simulink model "Project_microgrid"  (R2019b)
settings: Solver=FixedStepAuto  StartTime=0.0  StopTime=0.3  RelTol=1e-3
undefined symbols (not defined in the file): D1, D11, Delta, DiscIntNeverNeededParam, find_system, Hydride, Metal, Nickel
libraries: powerlib x108, powerlib_meascontrol x31, sps_avr x14, simulink_extras x4, simulink x3, spsDieselMotorModel x2, electricdrivelib x1, re_lib x1
(part 1 of 5)
settings Model: Creator=mdeat  LastModifiedBy=md ether
settings OptimizationCC: DefaultParameterBehavior=Inlined  EnhancedBackFolding=on  PassReuseOutputArgsAs=Individual arguments  ZeroExternalMemoryAtStartup=off  ZeroInternalMemoryAtStartup=off  MaxStackSize=64  OptimizeBlockOrder=speed  DifferentSizesBufferReuse=on  OptimizationCustomize=off  EfficientTunableParamExpr=on
settings DebuggingCC: ParameterTunabilityLossMsg=error
settings HardwareCC: ProdBitPerPointer=32  ProdBitPerSizeT=32  ProdBitPerPtrDiffT=32  ProdLargestAtomicInteger=Long  ProdLargestAtomicFloat=Double  ProdWordSize=32  ProdHWDeviceType=ARM Compatible->ARM Cortex
settings SFSimCC: MATLABDynamicMemAlloc=off  CustomCodeUndefinedFunction=UseInterfaceOnly
settings RTWCC: SystemTargetFile=ert.tlc  TemplateMakefile=ert_default_tmf  GenerateReport=on  Toolchain=Android SDK/NDK Tools  IncludeHyperlinkInReport=on  LaunchReport=on  GenerateTraceInfo=on  GenerateTraceReport=on  GenerateTraceReportSl=on  GenerateTraceReportSf=on  GenerateTraceReportEml=on
settings CodeAppCC: ForceParamTrailComments=on  IgnoreCustomStorageClasses=off  OperatorAnnotations=on  SimulinkDataObjDesc=on  SFDataObjDesc=on  InsertBlockDesc=on
settings ERTTargetCC: SupportContinuousTime=on  InlinedParameterPlacement=NonHierarchical  ERTCustomFileTemplate=example_file_process.tlc

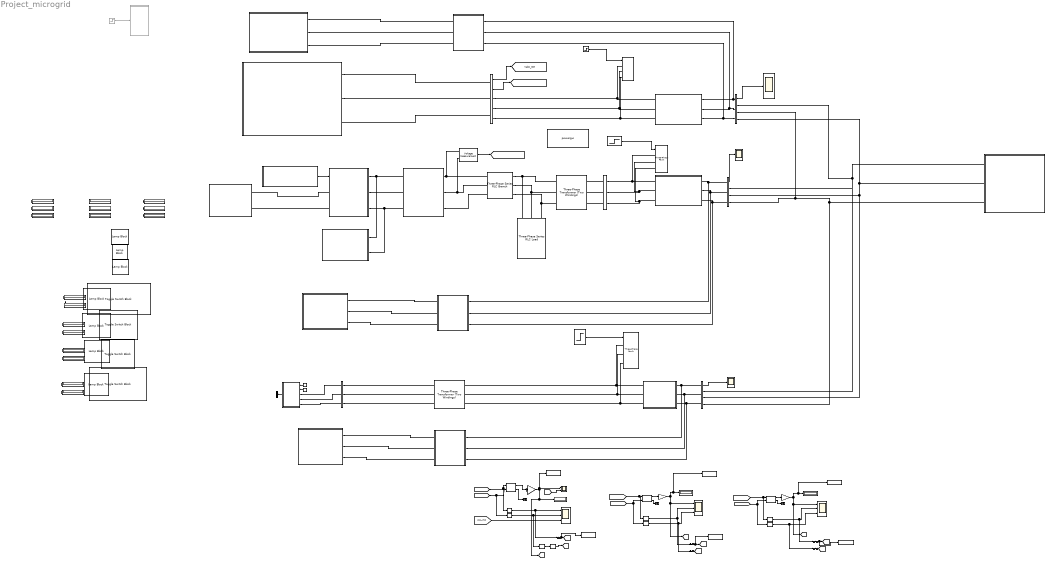
== system Project_microgrid ==
  note: Diesle Generator Output
  note: Wind Plant Output
  note: PV Output
  note: Fault Status
  note: Solar Power
  note: Solar Voltage
  note: Gen. Voltage
  note: Wind Power
  note: Gen. Current
  note: Current Power Status
  note: Gen. Power
  note: Solar Current
  note: Wind Current
  note: Wind Voltage
  note: PV Bus Fault
  note: Wind Bus Fault
  note: Generator Bus Fault
  note: Branch Status in Grid System
  note: Bus 1 Current
  note: Bus 1 Voltage
  note: Bus 2 Current
  note: Bus 2 Voltage
  note: Bus 3 Current
  note: Bus 3 Voltage
  note: Bus 4 Current
  note: Bus 4 Voltage
  " 2.2MWGenerator Backup" : Subsystem
  10 kvar Filter : powerlib/Elements/Three-Phase Series RLC Load  LConnTagsString=A|B|C  Configuration=Y (grounded)  NominalVoltage=240  Vabc=[1e3 1e3 1e3]  Vabcp=[1e3 1e3 1e3]  NominalFrequency=50  UnbalancedPower=off  ActivePower=10e3/100  InductivePower=0  CapacitivePower=10e3  Pabc=[10e3 9e3 11e3]  QLabc=[100 90 110]  QCabc=[100 90 110]  Pabcp=[10e3 9e3 11e3]  QLabcp=[100 90 110]  QCabcp=[100 90 110]  Measurements=None  LoadType=constant Z  mask(Three-Phase Series RLC Load){}
      settings: SourceProductName=Simscape Electrical
  100KW PV Backup : Subsystem
  260V / 25 kV : powerlib/Elements/Three-Phase Transformer (Two Windings)  Winding1Connection=Yg  Winding2Connection=Delta (D1)  CoreType=Three single-phase transformers  SetSaturation=off  Hysteresis=off  DataFile='hysteresis'  SetInitialFlux=off  Measurements=None  UNITS=pu  NominalPower=[7500 , 50 ]  Winding1=[ 25e3 , 0.001 , 0.03 ]  Winding2=[ 260 , 0.001 , 0.03 ]  Rm=500  Lm=500  L0=0.5  Saturation=[ 0,0 ; 0.0024,1.2 ; 1.0,1.52 ]  InitialFluxes=[ 0.8 , -0.8 , 0.7 ]  BreakLoop=off  DiscreteSolver=Trapezoidal iterative  DataType=off  TransfoNumber=0  mask(Three-Phase Transformer (Two Windings)){}
      settings: SourceProductName=Simscape Electrical
  "575 V/ 25 kV " : powerlib/Elements/Three-Phase Transformer (Two Windings)  Winding1Connection=Delta (D11)  Winding2Connection=Yg  CoreType=Three single-phase transformers  SetSaturation=off  Hysteresis=off  DataFile='hysteresis'  SetInitialFlux=off  Measurements=None  UNITS=pu  NominalPower="[2.5e6*5  60]"  Winding1=[25e3 , 0.025/30 , 0.025]  Winding2=[ 575, 0.025/30 , 0.025]  Rm=500  Lm=inf  L0=0.5  Saturation=[ 0,0 ; 0.0024,1.2 ; 1.0,1.52 ]  InitialFluxes=[ 0.8 , -0.8 , 0.7 ]  BreakLoop=off  DiscreteSolver=Trapezoidal iterative  DataType=off  TransfoNumber=0  mask(Three-Phase Transformer (Two Windings)){}
      settings: SourceProductName=Simscape Electrical
  600 KW Wind Backup2 : Subsystem
  Battery : Subsystem
  "Boost Conveter " : Subsystem
  Bus Selector : BusSelector  OutputSignals=Vdc_V,wr_pu,PQ_pu.P_pu,PQ_pu.Q_pu
  Constant : Constant  Value=15
  Constant1 : Constant  Value=0
  "Diesel Generator Bus " : powerlib/Measurements/Three-Phase V-I Measurement  VoltageMeasurement=phase-to-ground  SetLabelV=off  LabelV=Vabc  Vpu=off  VpuLL=off  CurrentMeasurement=yes  SetLabelI=off  LabelI=Iabc  Ipu=off  Pbase=100e6  Vbase=500e3  OutputType=Complex  PhasorSimulation=off  PSBequivalent=0
      settings: SourceProductName=Simscape Electrical
  Diesel Generator Bus 1 : powerlib/Measurements/Three-Phase V-I Measurement  VoltageMeasurement=no  SetLabelV=off  LabelV=Vabc  Vpu=off  VpuLL=off  CurrentMeasurement=yes  SetLabelI=off  LabelI=Iabc  Ipu=off  Pbase=100e6  Vbase=500e3  OutputType=Complex  PhasorSimulation=off  PSBequivalent=0
      settings: SourceProductName=Simscape Electrical
  Diesle Generator : Subsystem
  Grid : Scope  NumInputPorts=3
  Grid System : Subsystem
  Grid1 : Scope  NumInputPorts=3
  Grid2 : Scope  NumInputPorts=3
  Inveter : Subsystem
  Lamp{,1..6} (7 alike) : LampBlock
  MATLAB Function : MATLAB Function  Commented=on  TreatAsAtomicUnit=on
  "MPPT Controler " : Subsystem
  P (kW){,1..19} (20 alike) : Display
      settings: Format=bank  Decimation=2000
  PV Bus : powerlib/Measurements/Three-Phase V-I Measurement  VoltageMeasurement=phase-to-ground  SetLabelV=on  LabelV=Vabc_PV  Vpu=off  VpuLL=off  CurrentMeasurement=yes  SetLabelI=on  LabelI=Iabc_PV  Ipu=off  Pbase=100e6  Vbase=500e3  OutputType=Magnitude  PhasorSimulation=off  PSBequivalent=0
      settings: SourceProductName=Simscape Electrical
  PV Bus 1 : powerlib/Measurements/Three-Phase V-I Measurement  VoltageMeasurement=phase-to-ground  SetLabelV=off  LabelV=Vabc  Vpu=off  VpuLL=off  CurrentMeasurement=no  SetLabelI=off  LabelI=Iabc  Ipu=off  Pbase=100e6  Vbase=500e3  OutputType=Complex  PhasorSimulation=off  PSBequivalent=0
      settings: SourceProductName=Simscape Electrical
  "PV System " : Subsystem
  P_B1 : Scope  NumInputPorts=2
  Power (Positive-Sequence) : powerlib_meascontrol/Measurements/Power (Positive-Sequence)  Freq=60  Vinit=[0, 0]  Iinit=[0, 0]  Ts=0.0001
      settings: SourceProductName=Simscape Electrical  SourceProductBaseCode=PS
  Power (Positive-Sequence)1 : powerlib_meascontrol/Measurements/Power (Positive-Sequence)  Freq=60  Vinit=[0, 0]  Iinit=[0, 0]  Ts=0.0001
      settings: SourceProductName=Simscape Electrical  SourceProductBaseCode=PS
  Power (Positive-Sequence)2 : powerlib_meascontrol/Measurements/Power (Positive-Sequence)  Freq=60  Vinit=[0, 0]  Iinit=[0, 0]  Ts=0.0001
      settings: SourceProductName=Simscape Electrical  SourceProductBaseCode=PS
  Relay G : Subsystem
  Relay PV : Subsystem
  Relay W : Subsystem
  Scope2 : Scope
  Scope3 : Scope
  Scope4 : Scope
  Selector{,1..5} (6 alike) : Selector  InputPortWidth=3  IndexOptions=Index vector (dialog)  Indices=[1]  OutputSizes=1
  Sqrt{,1..5} (6 alike) : Sqrt  SaturateOnIntegerOverflow=on
  Square{,1..5} (6 alike) : Math  Operator=square  SignedPower=off  SaturateOnIntegerOverflow=on
  Step : Step  Commented=on  Time=0.5  After=5  SampleTime=0
  Step1 : Step  Time=0.25  SampleTime=0
  Step2 : Step  Time=0.05  SampleTime=0
  Step3 : Step  Time=0.2  SampleTime=0
  Switching Sustem : Subsystem
  Switching Sustem1 : Subsystem
  Switching Sustem3 : Subsystem
  TX Line Parameter : powerlib/Elements/Three-Phase Series RLC Branch  LConnTagsString=A|B|C  RConnTagsString=A|B|C  BranchType=RL  Resistance=500e-6*377/50/2  Inductance=500e-6/2  Capacitance=inf  Measurements=None
      settings: SourceProductName=Simscape Electrical
  Terminator1 : Terminator
  Terminator2 : Terminator
  Terminator3 : Terminator
  Three-Phase Fault1 : powerlib/Elements/Three-Phase Fault  InitialStates=[0 0 0]  FaultA=on  FaultB=on  FaultC=on  GroundFault=on  SwitchTimes="[1/60  5/60]"  External=on  SwitchStatus=NaN  FaultResistance=0.1  GroundResistance=0.01  SnubberResistance=1e6  SnubberCapacitance=inf  Measurements=None
      settings: SourceProductName=Simscape Electrical
  Three-Phase Fault2 : powerlib/Elements/Three-Phase Fault  InitialStates=[0 0 0]  FaultA=on  FaultB=on  FaultC=on  GroundFault=on  SwitchTimes="[1/60  5/60]"  External=on  SwitchStatus=NaN  FaultResistance=0.1  GroundResistance=0.01  SnubberResistance=1e6  SnubberCapacitance=inf  Measurements=None
      settings: SourceProductName=Simscape Electrical
  Three-Phase Fault3 : powerlib/Elements/Three-Phase Fault  InitialStates=[0 0 0]  FaultA=on  FaultB=on  FaultC=on  GroundFault=on  SwitchTimes="[1/60  5/60]"  External=on  SwitchStatus=NaN  FaultResistance=0.1  GroundResistance=0.01  SnubberResistance=1e6  SnubberCapacitance=inf  Measurements=None
      settings: SourceProductName=Simscape Electrical
  To Workspace : ToWorkspace  VariableName=PV_P  SaveFormat=Timeseries  SampleTime=-1
  To Workspace1 : ToWorkspace  VariableName=PV_V  SaveFormat=Timeseries  SampleTime=-1
  To Workspace2 : ToWorkspace  VariableName=W_P  SaveFormat=Timeseries  SampleTime=-1
  To Workspace3 : ToWorkspace  VariableName=W_V  SaveFormat=Timeseries  SampleTime=-1
  To Workspace4 : ToWorkspace  VariableName=G_P  SaveFormat=Timeseries  SampleTime=-1
  To Workspace5 : ToWorkspace  VariableName=G_V  SaveFormat=Timeseries  SampleTime=-1
  Toggle Switch{,1..3} (4 alike) : ToggleSwitchBlock
      settings: Values={{'Off', 'On'}, [0 1]}
  Vdc 1 : powerlib/Measurements/Voltage Measurement  Tag=PoWeRsYsTeMmEaSuReMeNt  PhasorSimulation=off  OutputType=Magnitude  PSBequivalent=0
      settings: SourceProductName=Simscape Electrical
  W : Gain  Gain=1/1000
  W1 : Gain  Gain=33.44
  W2kW : Gain  Gain=1/1000
  W2kW1 : Gain  Gain=1/1000
  Wind Bus : powerlib/Measurements/Three-Phase V-I Measurement  VoltageMeasurement=phase-to-ground  SetLabelV=on  LabelV=Vabc_Wind  Vpu=off  VpuLL=off  CurrentMeasurement=yes  SetLabelI=on  LabelI=Iabc_Wind  Ipu=off  Pbase=5*2e6/0.9  Vbase=575  OutputType=Complex  PhasorSimulation=off  PSBequivalent=0
      settings: SourceProductName=Simscape Electrical
  Wind Bus 1 : powerlib/Measurements/Three-Phase V-I Measurement  VoltageMeasurement=phase-to-ground  SetLabelV=off  LabelV=Vabc  Vpu=off  VpuLL=off  CurrentMeasurement=no  SetLabelI=off  LabelI=Iabc  Ipu=off  Pbase=100e6  Vbase=500e3  OutputType=Complex  PhasorSimulation=off  PSBequivalent=0
      settings: SourceProductName=Simscape Electrical
  Wind Turbine Type 4 : Subsystem  LoadFcn=%find_system(gcs,'FollowLinks', 'on', 'LookUnderMasks', 'all');  mask(Wind Turbine: Model 7){Nb_wt=5, ShowParameters=Generator data for 1 wind turbine, nom=[2e6/0.9 730 60], Reactances=[ 1.305, 0.296, 0.252, 0.474,  0.243,  0.18 ], Time_constants=[  4.49  0.0681  0.0513  ], Resistance=0.006, mec=[0.62 0.01 1], init=[ 0  0  0  0  0  0  0  0  1 ], Vnom=575, Imax_grid_conv=1.1, RL_grid=[ 0.15 0.15/50], C_var_filter1=150e3, Vdc_nom=1100, C_DClink1=90000e-6, L_R_Boost=[0.0012     5e-3], Pmec1=2e6, wind_speed_CpMax=11, wind0=11, DisplayTurbChar=off, H_WT=4.32, Ksh=0.3, D_mutual=1.5, w_wt0=1, torque0=1, Kdc=[1.1   27.5], Ki_var_reg=0.05, Ki_volt_reg=2, Kgrid_side_cur_reg=[1  50], Kspeed=[5 1], Kboost_cur_reg=[0.025 100], Kp_pitch=15, Kcompensation=[1.5  6], Kfield=[10  20], pitch_max=27, pitch_rate=10, Ts=2e-6}
      mask prompts: Nb_wt "Number of wind turbines:"; ShowParameters "Display:"; nom "Nom. power, L-L volt. and freq.: [Pn (VA), Vn (Vrms), fn (Hz)]"; Reactances "Reactances [Xd Xd' Xd'' Xq Xq'' Xl] (p.u.):"; Time_constants "Time constants [Tdo' Tdo'' Tq''] (s):"; Resistance "Resistance Rs (p.u.):"; mec "Inertia constant, friction factor, and pairs of poles: [ H(s)  F(p.u.)  p ]"; init "Initial conditions: [dw(%) th(deg) ia,ib,ic(pu) pha,phb,phc(deg) Vf(pu)]:"; Vnom "Grid-side converter nominal AC voltage (V):"; Imax_grid_conv "Grid-side converter maximum AC current (pu based on generator power and converter nominal AC voltage):"; RL_grid "Grid-side coupling inductor [ L(pu) R(pu),pu based on generator power and converter nominal AC voltage] :"; C_var_filter1 "Line filter capacitor (Q=50) (var):"; Vdc_nom "Nominal DC bus voltage (V)"; C_DClink1 "DC bus capacitor (F):"; L_R_Boost "Boost converter inductance [L(H) R(ohm)]:"; Pmec1 "Nominal mechanical output power (W):"; wind_speed_CpMax "Wind speed at nominal speed and at Cp max (must be between 6 m/s and 30 m/s) (m/s):"; wind0 "Initial wind speed (m/s):"; DisplayTurbChar "Display wind turbine power characteristics:"; H_WT "Wind turbine inertia constant H (s):"; Ksh "Shaft spring constant refer to high-speed shaft (pu of nominal mechanical torque/rad):"; D_mutual "Shaft mutual damping (pu of nominal mechanical torque/pu dw):"; w_wt0 "Turbine initial speed (pu of nominal speed):"; torque0 "Initial output torque (pu of nominal mechanical torque):"; Kdc "DC bus voltage regulator gains [Kp Ki]:"; Ki_var_reg "Grid-side converter var regulator gain [ Ki]:"; Ki_volt_reg "Grid-side converter voltage regulator gain [ Ki]:"; Kgrid_side_cur_reg "Grid-side converter current regulator gains [Kp Ki]:"; Kspeed "Speed regulator gains [Kp Ki]:"; Kboost_cur_reg "Boost inductor current regulator gains [Kp Ki]:"; Kp_pitch "Pitch controller gain [Kp]:"; Kcompensation "Pitch compensation gains [Kp Ki]:"; Kfield "Field excitation gains [Kp Ki]:"; pitch_max "Maximum pitch angle (deg):"; pitch_rate "Maximum rate of change of pitch angle (deg/s)"; Ts "Sample time (s):"
      mask help: This block implements a model of a variable speed pitch controlled wind turbine using a synchronous generator.
      mask init:
      | %Generator data
      | Pnom=nom(1)*Nb_wt;
      | Vnom_gen=nom(2);
      | Fnom=nom(3);
      | Xd=Reactances(1);
      | Xd1=Reactances(2);
      | Xd2=Reactances(3);
      | Xq=Reactances(4);
      | Xq2=Reactances(5);
      | Xl=Reactances(6);
      | Tdo1=Time_constants(1);
      | Tdo2=Time_constants(2);
      | Tq2=Time_constants(3);
      | H=mec(1);
      | F=mec(2);
      | p=mec(3);
      | 
      | % Converters data
      | L_RL=RL_grid(1);
      | R_RL=RL_grid(2);
      | L_Boost=L_R_Boost(1)/Nb_wt;
      | R_Boost=L_R_Boost(2)/Nb_wt;
      | Q_filter=50;
      | C_DClink=C_DClink1*Nb_wt;
      | C_var_filter=C_var_filter1*Nb_wt;
      | 
      | % Controller data
      | Freq_filter=10000;   %Hz
      | Zeta_filter=0.707;
      | Kp_dc=Kdc(1);
      | Ki_dc=Kdc(2);
      | Kp_grid_side_cur_reg=Kgrid_side_cur_reg(1);
      | Ki_grid_side_cur_reg=Kgrid_side_cur_reg(2);
      | Kp_speed=Kspeed(1);
      | Ki_speed=Kspeed(2);
      | Kp_boost_cur_reg=Kboost_cur_reg(1);
      | Ki_boost_cur_reg=Kboost_cur_reg(2);
      | Kp_compensation=Kcompensation(1);
      | Ki_compensation=Kcompensation(2);
      | Kp_field=Kfield(1);
      | Ki_field=Kfield(2);
      | Mod_index_max=1.1;
      | T_speed=5;      %Speed reference time constant (s)
      | Iq_ref_limit_time_constant=0.3; %(s)
      | Current_reg_output_limit=1.1;   %(pu)
      | Var_reg_output_hi_limit=1.1;    %(pu)
      | Var_reg_output_low_limit=0.9;   %(pu)
      | Pitch_time_constant=0.01;       %(s)
      | Vf_limit=10;    %Field voltage limit (pu)
      | Flux_meas_time_constant=1*(1/Fnom); %(s)
      | Freq_sawtooth=2000; %Hz, Boost converter
      | Freq_PWM=3000; %Hz, Inverter
      | Ts_snub=50e-6;  %Sample time to compute snubber resistance
      | 
      | 
      | % Turbine data
      | Pmec=Pmec1*Nb_wt;
      | c1 = 0.6450;
      | c2 = 116;
      | c3 = .4;
      | c4 = 5;
      | c5 = 21;
      | c6 = .00912;  % Set Pmin in stall condition (does not vary with wind_speed_Pmax)
      | c7 = .08;
      | c8 = .035;
      | theta=0;
      | CpMax=.5;
      | lambda_CpMax=9.9495;
      | 
      | c1_c8=[c1 c2 c3 c4 c5 c6 c7 c8];
      |   
      | 
      | %   Cp = c1*(c6*lambda + (-c4 - c3*(2.5 + theta) + c2*(1/(lambda + ...
      | %   c7*(2.5 + theta)) - c8/(1 + (2.5 + theta)^3)))/exp(c5*(1/(lambda + ...
      | %   c7*(2.5 + theta)) - c8/(1 + (2.5 + theta)^3))))
      | 
      | 
      |         %%%%%%%%%%%%%%%%%%%%%%%%%%%%%%%%%%%%%%%%%%%%%%%%%%%%%%%%%%%%%%%%%%%%%%%%%%%
      |         % Operation at Cp max
      |         %%%%%%%%%%%%%%%%%%%%%%%%%%%%%%%%%%%%%%%%%%%%%%%%%%%%%%%%%%%%%%%%%%%%%%%%%%%
      |         
      |         rated_omegar=1;
      |         omegar = rated_omegar;
      |         
      |         % Enforce boundaries on wind speed
      |         % A warning could be displayed
      |         if wind_speed_CpMax < 6
      |             wind_speed_CpMax=6;
      |             disp('Warning: Wind speed at nominal speed and at Cp max has been set to 6 m/s')
      |         end
      |         if wind_speed_CpMax > 30
      |             wind_speed_CpMax=30;
      |             disp('Warning: Wind speed at nominal speed and at Cp max has been set to 30 m/s')
      |         end
      | 
      |         K1=lambda_CpMax/omegar*wind_speed_CpMax;
      |         
      |         % Calculation of K2 needed to get P equal to the requested value at
      |         % Cp max for the requested wind speed
      |         
      |         Prated=Pmec;
      |         P_rated_omegar_theta_zero=0.75;
      |         
      |         K2 = P_rated_omegar_theta_zero*Prated/(wind_speed_CpMax^3*CpMax);
      |         
      |         K1_K2=[K1 K2];
      |         
      |         %%%%%%%%%%%%%%%%%%%%%%%%%%%%%%%%%%%%%%%%%%%%%%%%%%%%%%%%%%%%%%%%%%%%%%%%%%%
      |         % End of calculation for operation at Cp max
      |         %%%%%%%%%%%%%%%%%%%%%%%%%%%%%%%%%%%%%%%%%%%%%%%%%%%%%%%%%%%%%%%%%%%%%%%%%%%
      |         
      | 
      | %%%%%%%%%%%%%%%%%%%%%%%%%%%%%%%%%%%%%%%%%%%%%%%%%%%%%%%%%%%%%%%%%%%%%%%%%%%
      | % Plot turbine characteristics
      | %%%%%%%%%%%%%%%%%%%%%%%%%%%%%%%%%%%%%%%%%%%%%%%%%%%%%%%%%%%%%%%%%%%%%%%%%%% 
      | 
      | DisplayTurbChar=get_param(gcb,'DisplayTurbChar');
      | if strcmp(DisplayTurbChar,'on')
      |     vect_theta = 0:2:30;
      |     
      |     vect_lambda = 1:0.2:30;
      |     
      |     clear Cp;
      |     
      |     for i=1:length(vect_theta)
      |      for j=1:length(vect_lambda)
      |                 Cp(i,j) = c1*(c6*vect_lambda(j) + (-c4 - c3*(2.5 + vect_theta(i)) + c2*(1/(vect_lambda(j) + ...
      |                 c7*(2.5 + vect_theta(i))) - c8/(1 + (2.5 + vect_theta(i))^3)))/exp(c5*(1/(vect_lambda(j) + ...
      |                 c7*(2.5 + vect_theta(i))) - c8/(1 + (2.5 + vect_theta(i))^3))));
      |      end
      |     end
      | 
      |     figure(1);
      |     clf;
      |     hold on;
      | 
      |     plot(vect_lambda, Cp);
      |     axis([0, 25, 0, .6]);
      |     title('Wind Turbine Cp Characteristic (pitch angle increases by step of 2 deg.)');
      |     ylabel('Cp');
      |     set(gca,'ytick',[0 .1 .2 .3 .4 .5 .6]);
      |     xlabel('Lambda');
      |     grid on;
      |     text(10.1,0.51,'Pitch angle 0 degree');
      | 
      |     hold off
      |     
      |     % Plot of the wind turbine mechanical power output (pu) lambda and Cp
      |     % characteristics against wind speed (m/s) for a range of theta.
      |     
      |     wind_speed_range = [1,.2,30];
      |     vect_wind_speed = 1:0.2:30;
      |     
      |     clear lambda;
      |     clear Cp;
      |     clear P;
      | 
      |     for i=1:length(vect_theta)
      |         for j=1:length(vect_wind_speed)
      |             lambda(i,j) = K1*omegar/vect_wind_speed(j);
      |             Cp(i,j) = c1*(c6*lambda(i,j) + (-c4 - c3*(2.5 + vect_theta(i)) + c2*(1/(lambda(i,j) + ...
      |             c7*(2.5 + vect_theta(i))) - c8/(1 + (2.5 + vect_theta(i))^3)))/exp(c5*(1/(lambda(i,j) + ...
      |             c7*(2.5 + vect_theta(i))) - c8/(1 + (2.5 + vect_theta(i))^3))));
      |             P(i,j) = K2/Prated*vect_wind_speed(j)^3*Cp(i,j);
      |         end
      |     end
      |     
      |     
      |     figure(2);
      |     clf;
      |     hold on
      |     
      |     subplot(3,1,1);
      |     plot(vect_wind_speed, P);
      |     axis([0, 35, 0, 1.5]);
      |     title('Wind Turbine Characteristics (w = 1 pu, pitch angle increases by step of 2 deg.)');
      |     ylabel('P (pu)');
      |     set(gca,'ytick',0:.5:4);
      |     grid on;
      |     
      |     subplot(3,1,2);
      |     plot(vect_wind_speed, lambda);
      |     axis([0, 35, 0, 20]);
      |     ylabel('Lambda');
      |     grid on;
      |     
      |     subplot(3,1,3)
      |     plot(vect_wind_speed, Cp);
      |     axis([0, 35, 0, .6]);
      |     xlabel('Wind Speed (m/s)');
      |     ylabel('Cp');
      |     set(gca,'ytick',[0 .1 .2 .3 .4 .5 .6]);
      |     grid on;
      | 
      |     hold off
      |     set_param(gcb,'DisplayTurbChar','off')
      |     
      | end
      mask TypeOptions ShowParameters: Generator data for 1 wind turbine | Converters data for 1 wind turbine | Turbine data for 1 wind turbine | Drive train data for 1 wind turbine | Control parameters for 1 wind turbine
      mask Callback ShowParameters:
      | BlockName=getfullname(gcb);
      | %
      | Param_Show=get_param(BlockName,'ShowParameters');
      | Param_DisplayTurbChar=get_param(BlockName,'DisplayTurbChar');
      | 
      | p_mask{3}='off';p_mask{4}='off';p_mask{5}='off';
      | p_mask{6}='off';p_mask{7}='off';p_mask{8}='off';p_mask{9}='off';
      | p_mask{10}='off';p_mask{11}='off';p_mask{12}='off';p_mask{13}='off';
      | p_mask{14}='off';p_mask{15}='off';p_mask{16}='off';p_mask{17}='off';
      | p_mask{18}='off';p_mask{19}='off';p_mask{20}='off';p_mask{21}='off';
      | p_mask{22}='off';p_mask{23}='off';p_mask{24}='off';p_mask{25}='off';
      | p_mask{26}='off';p_mask{27}='off';p_mask{28}='off';p_mask{29}='off';
      | p_mask{30}='off';p_mask{31}='off';p_mask{32}='off';p_mask{33}='off';
      | p_mask{34}='off';p_mask{35}='off';
      | 
      | switch Param_Show
      | 	case 'Generator data for 1 wind turbine'
      | 		p_mask{3}='on';p_mask{4}='on';p_mask{5}='on';
      |         p_mask{6}='on';p_mask{7}='on';p_mask{8}='on';
      |     case 'Converters data for 1 wind turbine'
      | 		p_mask{9}='on';p_mask{10}='on';p_mask{11}='on';
      |         p_mask{12}='on';p_mask{13}='on';p_mask{14}='on';p_mask{15}='on';
      | 	case 'Turbine data for 1 wind turbine'
      | 		p_mask{16}='on';p_mask{17}='on';p_mask{18}='on';p_mask{19}='on';
      |     case 'Drive train data for 1 wind turbine'
      |         p_mask{20}='on';p_mask{21}='on';p_mask{22}='on';p_mask{23}='on';
      |         p_mask{24}='on';
      |     case 'Control parameters for 1 wind turbine'
      |         p_mask{25}='on';p_mask{26}='on';p_mask{27}='on';
      |         p_mask{28}='on';p_mask{29}='on';p_mask{30}='on';p_mask{31}='on';
      |         p_mask{32}='on';p_mask{33}='on';p_mask{34}='on';p_mask{35}='on';
      | end
      | 
      | ParVisible={'on','on',p_mask{3},p_mask{4},p_mask{5},p_mask{6},...
      |     p_mask{7},p_mask{8},p_mask{9},p_mask{10},p_mask{11},p_mask{12},...
      |     p_mask{13},p_mask{14},p_mask{15},p_mask{16},p_mask{17},p_mask{18},...
      |     p_mask{19},p_mask{20},p_mask{21},p_mask{22},p_mask{23},p_mask{24},...
      |     p_mask{25},p_mask{26},p_mask{27},p_mask{28},p_mask{29},p_mask{30},...
      |     p_mask{31},p_mask{32},p_mask{33},p_mask{34},p_mask{35},'on'};
      | %
      | set_param(BlockName,'MaskVisibilities',ParVisible);
      | set_param(BlockName,'DisplayTurbChar',Param_DisplayTurbChar);
      mask Display: disp(' ');
  powergui : powerlib/powergui  Priority=1  SimulationMode=Discrete  SampleTime=4e-6  frequency=60  Iterations=50  frequencyindice=0  Pbase=100e6  ErrMax=1e-4  UnitsV=kV  UnitsW=MW  buscounter=0  FunctionMessages=off  echomessages=off  EnableUseOfTLC=off  CurrentSourceSwitches=off  DisableSnubberDevices=off  DisableRonSwitches=off  DisableVfSwitches=off  DisplayEquations=off  AutomaticDiscreteSolvers=off  SolverType=Tustin/Backward Euler (TBE)  Interpol=off  ExternalGateDelay=off  methode=off  Ts=0  x0status=blocks  SPID=off  SwTol=0  HookPort=off  NonlinearTolerance=0  nMaxIteration=15  ContinueOnMaxIteration=off  RestoreLinks=warning  ResistiveCurrentMeasurement=off  Frange=[0:2:500]  Ylog=off  Xlog=on  ShowGrid=off  save=off  variable=ZData  structure=0  ZoomFFT=on  StartTime=0.0  cycles=1  DisplayStyle=1  fundamental=60  FreqAxis=off  MaxFrequency=1000  frequencyindicesteady=1  RmsSteady=1  display=off
      settings: SourceProductName=Simscape Electrical
  tag scope: G_i=global, G_p=global, G_v=global, Iabc_DG=global, PV_i=global, PV_p=global, PV_v=global, Vab_VSC=global, Vabc_DG=global, W_i=global, W_p=global, W_v=global
  wires:
  "MPPT Controler "/1(Boost Conveter Pulse) -> "Boost Conveter "/1(Pulse)
  Vdc 1/1 -> [Vab_VSC]
  "Diesel Generator Bus "/2 -> [Iabc_DG]
  "Diesel Generator Bus "/1 -> [Vabc_DG]
  Step1/1 -> Three-Phase Fault1/1  "Wind Fault"
  Step2/1 -> Three-Phase Fault2/1  "Generator Fault"
  Step3/1 -> Three-Phase Fault3/1  "PV Fault"
  Diesel Generator Bus 1/1 -> Scope2/1  "Diesel Generator Bus"
  Wind Bus 1/1 -> Scope3/1  "Wind Bus"
  PV Bus 1/1 -> Scope4/1  "PV Bus"
  [Vdc] -> P_B1/2
  Selector/1 -> Square/1, Grid/1  "(V)"
  [Vab_VSC] -> Grid/3
  [Iabc_PV] -> Power (Positive-Sequence)/2, Selector1/1
  Power (Positive-Sequence)2/2 -> Terminator3/1
  [Iabc_DG] -> Power (Positive-Sequence)2/2, Selector5/1
  W2kW/1 -> [G_p], Grid2/1, To Workspace4/1, P (kW)2/1  "P (kW)"
  [Vabc_PV] -> Power (Positive-Sequence)/1, Selector/1
  Selector1/1 -> Square1/1, Grid/2  "Ia (A)"
  Power (Positive-Sequence)/2 -> Terminator1/1
  Power (Positive-Sequence)2/1 -> W2kW/1
  Selector4/1 -> Square4/1, Grid2/2  "Va (V)"
  Selector5/1 -> Square5/1, Grid2/3  "Ia (A)"
  Selector3/1 -> Square3/1, Grid1/3  "Ia (A)"
  Power (Positive-Sequence)1/1 -> W2kW1/1
  W2kW1/1 -> [W_p], Grid1/1, To Workspace2/1, P (kW)1/1  "P (kW)"
  [Iabc_Wind] -> Power (Positive-Sequence)1/2, Selector3/1
  Power (Positive-Sequence)1/2 -> Terminator2/1
  [Vabc_Wind] -> Power (Positive-Sequence)1/1, Selector2/1
  W/1 -> [PV_p], P (kW)/1, To Workspace/1, P_B1/1  "P (kW)"
  [Vabc_DG] -> Power (Positive-Sequence)2/1, Selector4/1
  Constant1/1 -> Wind Turbine Type 4/2(Qref_pu)
  Constant/1 -> Wind Turbine Type 4/1("Wind (m/s) ")
  Wind Turbine Type 4/1(m) -> Bus Selector/1
  W1/1 -> W/1  "P (kW)"
  Power (Positive-Sequence)/1 -> W1/1
  [W_p] -> P (kW)6/1
  [PV_i] -> P (kW)5/1
  [W_v] -> P (kW)7/1
  [PV_v] -> P (kW)4/1
  [G_i] -> P (kW)11/1
  [G_p] -> P (kW)9/1
  [W_i] -> P (kW)8/1
  [PV_p] -> P (kW)3/1
  [G_v] -> P (kW)10/1
  [vabc_3] -> P (kW)12/1
  [iabc_6] -> P (kW)15/1
  [vabc_6] -> P (kW)14/1
  [iabc_9] -> P (kW)17/1
  [vabc_9] -> P (kW)16/1
  [iabc_11] -> P (kW)19/1
  [vabc_11] -> P (kW)18/1
  Sqrt/1 -> To Workspace1/1, [PV_v]
  Square/1 -> Sqrt/1
  Sqrt1/1 -> [PV_i]
  Square1/1 -> Sqrt1/1
  Selector2/1 -> Square2/1, Grid1/2  "Va (V)"
  Square2/1 -> Sqrt2/1
  Sqrt2/1 -> To Workspace3/1, [W_v]
  Square3/1 -> Sqrt3/1
  Sqrt3/1 -> [W_i]
  Square4/1 -> Sqrt4/1
  Sqrt4/1 -> To Workspace5/1, [G_v]
  Square5/1 -> Sqrt5/1
  Sqrt5/1 -> [G_i]
  Step/1 -> MATLAB Function/1(b)
  connections:
  "Boost Conveter "/RConn1 -- Battery/RConn1 -- Inveter/RConn1
  "Boost Conveter "/RConn2 -- Inveter/RConn2
  "Boost Conveter "/RConn3 -- Battery/RConn2 -- Inveter/RConn3
  "Boost Conveter "/LConn1 -- "PV System "/RConn1
  "Boost Conveter "/LConn2 -- "PV System "/RConn2
  Wind Bus/LConn1 -- "575 V/ 25 kV "/RConn1
  Wind Bus/LConn3 -- "575 V/ 25 kV "/RConn3
  Wind Bus/LConn2 -- "575 V/ 25 kV "/RConn2
  Inveter/LConn2 -- Vdc 1/LConn2 -- TX Line Parameter/LConn2
  TX Line Parameter/RConn2 -- 260V / 25 kV/RConn2 -- 10 kvar Filter/LConn2
  TX Line Parameter/RConn1 -- 10 kvar Filter/LConn1 -- 260V / 25 kV/RConn1
  TX Line Parameter/RConn3 -- 10 kvar Filter/LConn3 -- 260V / 25 kV/RConn3
  Inveter/LConn1 -- Vdc 1/LConn1 -- TX Line Parameter/LConn1
  Inveter/LConn3 -- TX Line Parameter/LConn3
  PV Bus/LConn3 -- 260V / 25 kV/LConn3
  PV Bus/LConn1 -- 260V / 25 kV/LConn1
  PV Bus/LConn2 -- 260V / 25 kV/LConn2
  "Diesel Generator Bus "/LConn3 -- Diesle Generator/RConn3
  Diesle Generator/RConn2 -- "Diesel Generator Bus "/LConn2
  Diesle Generator/RConn1 -- "Diesel Generator Bus "/LConn1
  Relay W/RConn1 -- Three-Phase Fault1/LConn1 -- "575 V/ 25 kV "/LConn1
  Relay W/RConn3 -- Three-Phase Fault1/LConn3 -- "575 V/ 25 kV "/LConn3
  Relay W/RConn2 -- Three-Phase Fault1/LConn2 -- "575 V/ 25 kV "/LConn2
  Three-Phase Fault2/LConn1 -- Relay G/RConn1 -- "Diesel Generator Bus "/RConn1
  "Diesel Generator Bus "/RConn2 -- Three-Phase Fault2/LConn2 -- Relay G/RConn2
  "Diesel Generator Bus "/RConn3 -- Three-Phase Fault2/LConn3 -- Relay G/RConn3
  Three-Phase Fault3/LConn1 -- Relay PV/RConn1 -- PV Bus/RConn1
  PV Bus/RConn2 -- Three-Phase Fault3/LConn2 -- Relay PV/RConn2
  PV Bus/RConn3 -- Three-Phase Fault3/LConn3 -- Relay PV/RConn3
  Relay G/LConn1 -- Switching Sustem/RConn1 -- Diesel Generator Bus 1/LConn1
  Relay G/LConn2 -- Switching Sustem/RConn2 -- Diesel Generator Bus 1/LConn2
  Relay G/LConn3 -- Switching Sustem/RConn3 -- Diesel Generator Bus 1/LConn3
  Wind Bus 1/LConn1 -- Switching Sustem3/RConn1 -- Relay W/LConn1
  Wind Bus 1/LConn2 -- Switching Sustem3/RConn2 -- Relay W/LConn2
  Wind Bus 1/LConn3 -- Switching Sustem3/RConn3 -- Relay W/LConn3
  PV Bus 1/LConn1 -- Switching Sustem1/RConn1 -- Relay PV/LConn1
  Relay PV/LConn2 -- Switching Sustem1/RConn2 -- PV Bus 1/LConn2
  PV Bus 1/LConn3 -- Switching Sustem1/RConn3 -- Relay PV/LConn3
  Wind Turbine Type 4/LConn1 -- Wind Bus/RConn1
  Wind Turbine Type 4/LConn2 -- Wind Bus/RConn2
  Wind Turbine Type 4/LConn3 -- Wind Bus/RConn3
  " 2.2MWGenerator Backup"/RConn1 -- Switching Sustem/LConn1
  " 2.2MWGenerator Backup"/RConn2 -- Switching Sustem/LConn2
  " 2.2MWGenerator Backup"/RConn3 -- Switching Sustem/LConn3
  100KW PV Backup/RConn1 -- Switching Sustem1/LConn1
  100KW PV Backup/RConn2 -- Switching Sustem1/LConn2
  100KW PV Backup/RConn3 -- Switching Sustem1/LConn3
  Diesel Generator Bus 1/RConn3 -- Wind Bus 1/RConn2 -- PV Bus 1/RConn2 -- Grid System/LConn2
  Diesel Generator Bus 1/RConn2 -- Wind Bus 1/RConn3 -- Grid System/LConn3 -- PV Bus 1/RConn3
  Diesel Generator Bus 1/RConn1 -- Wind Bus 1/RConn1 -- PV Bus 1/RConn1 -- Grid System/LConn1
  600 KW Wind Backup2/RConn2 -- Switching Sustem3/LConn2
  600 KW Wind Backup2/RConn1 -- Switching Sustem3/LConn1
  600 KW Wind Backup2/RConn3 -- Switching Sustem3/LConn3

== system Project_microgrid/ 2.2MWGenerator Backup ==
  Diesel Generator Bus 2 : powerlib/Measurements/Three-Phase V-I Measurement  VoltageMeasurement=no  SetLabelV=off  LabelV=Vabc  Vpu=off  VpuLL=off  CurrentMeasurement=no  SetLabelI=off  LabelI=Iabc  Ipu=off  Pbase=100e6  Vbase=500e3  OutputType=Complex  PhasorSimulation=off  PSBequivalent=0
      settings: SourceProductName=Simscape Electrical
  Diesle Generator1 : Subsystem
  Conn1 : PMIOPort  Side=Right
  Conn2 : PMIOPort  Port=2  Side=Right
  Conn3 : PMIOPort  Port=3  Side=Right
  connections:
  Diesel Generator Bus 2/RConn2 -- Conn2/RConn1
  Diesel Generator Bus 2/LConn3 -- Diesle Generator1/RConn3
  Diesle Generator1/RConn2 -- Diesel Generator Bus 2/LConn2
  Diesle Generator1/RConn1 -- Diesel Generator Bus 2/LConn1
  Diesel Generator Bus 2/RConn1 -- Conn1/RConn1
  Diesel Generator Bus 2/RConn3 -- Conn3/RConn1

== system Project_microgrid/100KW PV Backup ==
  Three-Phase AC Source : powerlib/Electrical Sources/Three-Phase Source  InternalConnection=Yg  VoltagePhases=off  Voltage=25e3  PhaseAngle=0  Voltage_phases=[25e3 25e3 25e3]/sqrt(3)  PhaseAngles_phases=[0 -120 +120]  Frequency=60  NonIdealSource=on  SpecifyImpedance=off  Resistance=0.8929  Inductance=16.58e-3  ShortCircuitLevel=100e6  BaseVoltage=25e3  XRratio=7  BusType=swing  Pref=10e3  Qref=0  Prefabc=[10e3, 10e3, 10e3]  Qrefabc=[0, 0, 0]  Qmin=-inf  Qmax=inf
      settings: SourceProductName=Simscape Electrical
  Conn1 : PMIOPort  Side=Right
  Conn2 : PMIOPort  Port=2  Side=Right
  Conn3 : PMIOPort  Port=3  Side=Right
  connections:
  Three-Phase AC Source/RConn1 -- Conn1/RConn1
  Three-Phase AC Source/RConn3 -- Conn3/RConn1
  Three-Phase AC Source/RConn2 -- Conn2/RConn1

== system Project_microgrid/600 KW Wind Backup2 ==
  Three-Phase Source : powerlib/Electrical Sources/Three-Phase Source  InternalConnection=Yg  VoltagePhases=off  Voltage=25e3  PhaseAngle=0  Voltage_phases=[25e3 25e3 25e3]/sqrt(3)  PhaseAngles_phases=[0 -120 +120]  Frequency=60  NonIdealSource=on  SpecifyImpedance=off  Resistance=0.8929  Inductance=16.58e-3  ShortCircuitLevel=100e6  BaseVoltage=25e3  XRratio=7  BusType=swing  Pref=10e3  Qref=0  Prefabc=[10e3, 10e3, 10e3]  Qrefabc=[0, 0, 0]  Qmin=-inf  Qmax=inf
      settings: SourceProductName=Simscape Electrical
  Conn1 : PMIOPort  Side=Right
  Conn2 : PMIOPort  Port=2  Side=Right
  Conn3 : PMIOPort  Port=3  Side=Right
  connections:
  Three-Phase Source/RConn1 -- Conn1/RConn1
  Three-Phase Source/RConn3 -- Conn3/RConn1
  Three-Phase Source/RConn2 -- Conn2/RConn1

== system Project_microgrid/Battery ==
  Battery : electricdrivelib/Extra Sources/Battery  BatType=Nickel-Metal-Hydride  ShowTempParam=off  ThermalPreset=no  ShowAgeParam=off  NomV=220  NomQ=100  SOC=100  Batt_Tr=30  PresetModel=on  MaxQ=107.6923  MinV=165  FullV=259.1525  Dis_rate=20  R=0.022  Normal_OP=96.1538  expZone="[238.6441            20]"  current=[6.5 13 32.5]  Units=Time  Tci=20  NomT=20  T2=-30  MaxQ2=4.8  FullV2=7.1  Normal_OP2=5.655  expZone2="[6.58           1]"  Rca=0.6  ti=2000  Dp=0  Neq0=0  Tsim=1e6  Ta1=25  Qeol=5.4*0.9  Reol=0.013333*1.2  Char_age=[2.3478, 3]  Dis_age=[2.3478, 10]  N1=1500  N2=10500  N3=1000  N4=1400  Ta2=45  N5=950
      settings: SourceProductName=Simscape Electrical
  Bus Selector1 : BusSelector  OutputSignals=Current (A),Voltage (V)
  Scope3 : Scope  NumInputPorts=2
  Subsystem4 : Subsystem
      mask Display: disp('Converter')
  Conn1 : PMIOPort  Side=Right
  Conn2 : PMIOPort  Port=2  Side=Right
  wires:
  Bus Selector1/2 -> Scope3/2  "<Voltage (V)>"
  Bus Selector1/1 -> Scope3/1  "<Current (A)>"
  Battery/1 -> Bus Selector1/1
  connections:
  Battery/LConn1 -- Subsystem4/LConn1
  Subsystem4/RConn1 -- Conn1/RConn1
  Subsystem4/RConn2 -- Conn2/RConn1
  Battery/LConn2 -- Subsystem4/LConn2

== system Project_microgrid/Boost Conveter  ==
  Pulse : Inport
  C1 : powerlib/Elements/Series RLC Branch  LConnTagsString=__new0  RConnTagsString=__new0  BranchType=C  Resistance=1.0  Inductance=1.0  SetiL0=off  InitialCurrent=0  Capacitance=12000e-06  Setx0=off  InitialVoltage=0  Measurements=None
      settings: SourceProductName=Simscape Electrical
  C2 : powerlib/Elements/Series RLC Branch  LConnTagsString=__new0  RConnTagsString=__new0  BranchType=C  Resistance=1.0  Inductance=1.0  SetiL0=off  InitialCurrent=0  Capacitance=12000e-06  Setx0=off  InitialVoltage=0  Measurements=None
      settings: SourceProductName=Simscape Electrical
  C3 : powerlib/Elements/Series RLC Branch  LConnTagsString=__new0  RConnTagsString=__new0  BranchType=C  Resistance=1.0  Inductance=1.0  SetiL0=off  InitialCurrent=0  Capacitance=100e-6  Setx0=off  InitialVoltage=0  Measurements=Branch voltage
      settings: SourceProductName=Simscape Electrical
  Diode1 : powerlib/Power Electronics/Diode  Ron=1e-4  Lon=0  Vf=0  IC=0  UseSnubber=off  Rs=inf  Cs=inf  Measurements=off
      settings: SourceProductName=Simscape Electrical
  IGBT1 : powerlib/Power Electronics/IGBT  Ron=0.001  Lon=0  Vf=0  Tf=0  Tt=0  IC=0  Rs=1e5  Cs=inf  Measurements=off
      settings: SourceProductName=Simscape Electrical
  L1 : powerlib/Elements/Series RLC Branch  LConnTagsString=__new0  RConnTagsString=__new0  BranchType=RL  Resistance=0.005  Inductance=5e-3  SetiL0=off  InitialCurrent=0  Capacitance=1e-6  Setx0=off  InitialVoltage=0  Measurements=None
      settings: SourceProductName=Simscape Electrical
  "Vdc " : powerlib/Measurements/Voltage Measurement  Tag=PoWeRsYsTeMmEaSuReMeNt  PhasorSimulation=off  OutputType=Magnitude  PSBequivalent=0
      settings: SourceProductName=Simscape Electrical
  +Vin : PMIOPort  Side=Left
  +Vout : PMIOPort  Port=2  Side=Right
  N : PMIOPort  Port=3  Side=Right
  -Vout : PMIOPort  Port=4  Side=Right
  -Vin : PMIOPort  Port=5  Side=Left
  tag scope: Vdc=global
  wires:
  Pulse/1 -> IGBT1/1
  "Vdc "/1 -> [Vdc]
  connections:
  "Vdc "/LConn1 -- +Vout/RConn1 -- C1/LConn1 -- Diode1/RConn1
  C3/RConn1 -- -Vin/RConn1 -- IGBT1/RConn1 -- "Vdc "/LConn2 -- -Vout/RConn1 -- C2/RConn1
  IGBT1/LConn1 -- L1/RConn1 -- Diode1/LConn1
  C1/RConn1 -- N/RConn1 -- C2/LConn1
  C3/LConn1 -- +Vin/RConn1 -- L1/LConn1

== system Project_microgrid/Diesle Generator ==
  Bus Selector2 : BusSelector  OutputSignals="Mechanical.Rotor speed  wm  (pu)"  OutputAsBus=on
  Bus Selector4 : BusSelector  OutputSignals="dq0 components.Field current  ifd (pu)"  OutputAsBus=on
  Bus Selector5 : BusSelector  OutputSignals="dq0 components.Stator voltage  vd (pu),dq0 components.Stator voltage  vq (pu)"  OutputAsBus=on
  Bus Selector6 : BusSelector  OutputSignals="dq0 components.Stator current  id (pu),dq0 components.Stator current  iq (pu)"  OutputAsBus=on
  Diesel Engine Governor : spsDieselMotorModel/Diesel Engine Governor  K=40  Tr=[0.01 0.02 0.2]  Ta=[0.25 0.009 0.0384]  Tlim=[0 1.1]  Td=0.024  Pm0=0
      settings: SourceProductName=Simscape Electrical  SourceProductBaseCode=PS
  EXCITATION : Subsystem  VariantControlMode=Label  Variant=on  LabelModeActiveChoice=Variant1
      settings: AttributesFormatString=%<BlockChoice>
  Fcn1 : Fcn  Expr=sqrt(u(1)^2 + u(2)^2)
  Fcn2 : Fcn  Expr=sqrt(u(1)^2 + u(2)^2)
  Ground : Ground
  SM : Scope  NumInputPorts=4
  SM 3.125 MVA : powerlib/Machines/Synchronous Machine pu Standard  PresetModel=No  MechanicalLoad=Mechanical power Pm  ShowDetailedParameters=on  RotorType=Salient-pole  Units=per unit standard parameters  MeasurementBus=off  NominalParameters="[ 3.125e6  2400  60]"  Reactances1=[ 31 32 33 34 35 36 37 ]  Reactances2=[ 1.56, 0.296, 0.177, 1.06, 0.177, 0.052 ]  dAxisTimeConstants=Short-circuit  qAxisTimeConstants=Open-circuit  TimeConstants1=[]  TimeConstants2=[]  TimeConstants3=[]  TimeConstants4=[]  TimeConstants5=[ 3.7, 0.05, 0.05 ]  TimeConstants6=[ 8.0, 0.03, 0.3371, 0.0295 ]  TimeConstants7=[0.024 0.006 0.006]  TimeConstants8=[]  StatorResistance=0.0036  Mechanical="[ 1.07  0 2]"  PolePairs=2  InitialConditions=[0 0 0 0 0 0 0 0 1]  SetSaturation=off  Saturation=[0.211 0.418 1.0 1.25 1.72 3.35 ;0.25 0.50 1.0 1.1 1.2 1.4]  LoadFlowParameters=[1 0 0 0]  TsPowergui=0  TsBlock=-1  IterativeModel=Trapezoidal non iterative  IterativeDiscreteModel=Trapezoidal non iterative  BusType=PV  Pref=0  Qref=0  Qmin=-Inf  Qmax=Inf  PLF=0  QLF=0
      settings: AttributesFormatString=\n\n  SourceProductName=Simscape Electrical
  "Vtref (pu) " : Constant
  wref (pu) : Constant
  Conn1 : PMIOPort  Side=Right
  Conn2 : PMIOPort  Port=2  Side=Right
  Conn3 : PMIOPort  Port=3  Side=Right
  wires:
  Ground/1 -> EXCITATION/5(Vstab)  "Not implemented"
  Diesel Engine Governor/1 -> SM/2, SM 3.125 MVA/1  "Pm"
  SM 3.125 MVA/1 -> Bus Selector2/1, Bus Selector5/1, Bus Selector6/1, Bus Selector4/1
  Fcn2/1 -> EXCITATION/3(It)
  Fcn1/1 -> SM/4, EXCITATION/2(Vt)  "Vt"
  Bus Selector5/1 -> Fcn1/1  "Vd Vq"
  EXCITATION/1(Efd) -> SM/3, SM 3.125 MVA/2  "Vf"
  Bus Selector2/1 -> Diesel Engine Governor/2, SM/1  "Wm"
  wref (pu)/1 -> Diesel Engine Governor/1
  "Vtref (pu) "/1 -> EXCITATION/1(Vref)
  Bus Selector6/1 -> Fcn2/1  "Id Iq"
  Bus Selector4/1 -> EXCITATION/4(Ifd)  "Ifd"
  connections:
  Conn2/RConn1 -- SM 3.125 MVA/RConn2
  Conn3/RConn1 -- SM 3.125 MVA/RConn3
  Conn1/RConn1 -- SM 3.125 MVA/RConn1
